simulink model "lab_4_3_2016b"  (R2016b)
settings: Solver=VariableStepAuto  StartTime=0.0  StopTime=2  RelTol=1e-3
libraries: simulink x1
settings Model: Creator=kamzab95  LastModifiedBy=kamzab95

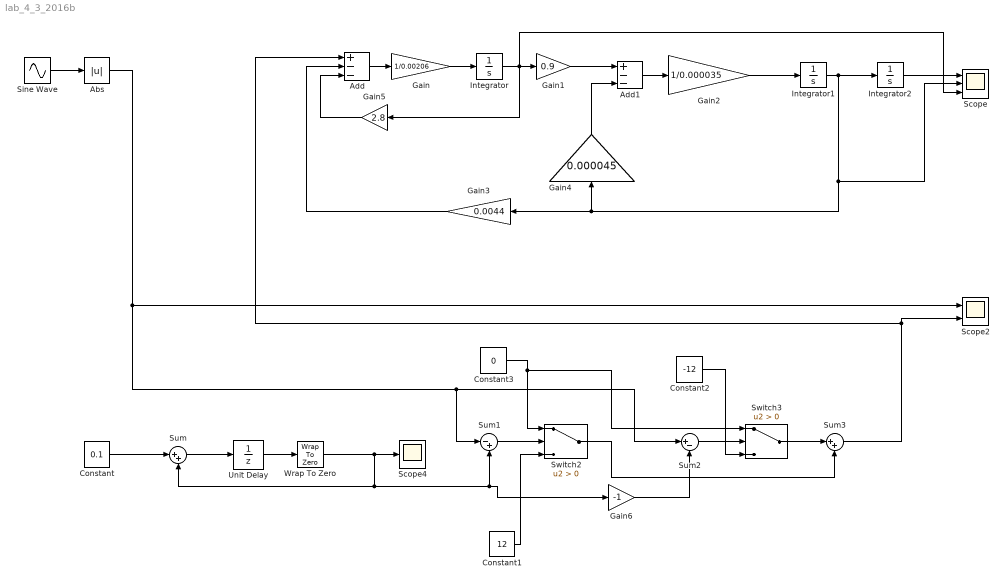
== system lab_4_3_2016b ==
  Abs : Abs
  Add : Sum  Inputs=+--
  Add1 : Sum  Inputs=+--
  Constant : Constant  Value=0.1
  Constant1 : Constant  Value=12
  Constant2 : Constant  Value=-12
  Constant3 : Constant  Value=0
  Gain : Gain  Gain=1/0.00206
  Gain1 : Gain  Gain=0.9
  Gain2 : Gain  Gain=1/0.000035
  Gain3 : Gain  Gain=0.0044
  Gain4 : Gain  Gain=0.000045
  Gain5 : Gain  Gain=2.8
  Gain6 : Gain  Gain=-1
  Integrator : Integrator
  Integrator1 : Integrator
  Integrator2 : Integrator
  Scope : Scope  NumInputPorts=3
  Scope2 : Scope  NumInputPorts=2
  Scope4 : Scope
  Sine Wave : Sin  Amplitude=12  Frequency=50  SampleTime=0
  Sum : Sum  Inputs=|++
  Sum1 : Sum  Inputs=|-+
  Sum2 : Sum  Inputs=|+-
  Sum3 : Sum  Inputs=|++
  Switch2 : Switch  Criteria=u2 > Threshold
  Switch3 : Switch  Criteria=u2 > Threshold
  Unit Delay : UnitDelay  SampleTime=0.00005
  Wrap To Zero : simulink/Discontinuities/Wrap To Zero  Threshold=12
  wires:
  Add/1 -> Gain/1
  Gain/1 -> Integrator/1
  Integrator/1 -> Gain5/1, Scope/3, Gain1/1
  Gain1/1 -> Add1/1
  Add1/1 -> Gain2/1
  Gain2/1 -> Integrator1/1
  Integrator1/1 -> Integrator2/1, Scope/2, Gain3/1, Gain4/1
  Gain3/1 -> Add/2
  Gain5/1 -> Add/3
  Gain4/1 -> Add1/3
  Integrator2/1 -> Scope/1
  Sine Wave/1 -> Abs/1
  Gain6/1 -> Sum2/2
  Sum2/1 -> Switch3/2
  Constant/1 -> Sum/1
  Constant2/1 -> Switch3/3
  Switch2/1 -> Sum3/2
  Wrap To Zero/1 -> Scope4/1, Sum/2, Gain6/1, Sum1/2
  Sum/1 -> Unit Delay/1
  Unit Delay/1 -> Wrap To Zero/1
  Constant1/1 -> Switch2/3
  Switch3/1 -> Sum3/1
  Constant3/1 -> Switch3/1, Switch2/1
  Sum1/1 -> Switch2/2
  Abs/1 -> Sum2/1, Sum1/1, Scope2/1
  Sum3/1 -> Add/1, Scope2/2
